simulink model "hil2DOFArmSynergyTemplate"  (R2017a)
settings: Solver=FixedStepAuto  StartTime=0.0  StopTime=5  RelTol=1e-3
undefined symbols (not defined in the file): alpha, armDynamics, get
libraries: vrlib x4, myo_lib x3, dspstat3 x2, aerolibconvert2 x1, sldrtlib x1
settings Model: Creator=ricardog  LastModifiedBy=ricardog
settings SolverCC: AutoInsertRateTranBlk=on

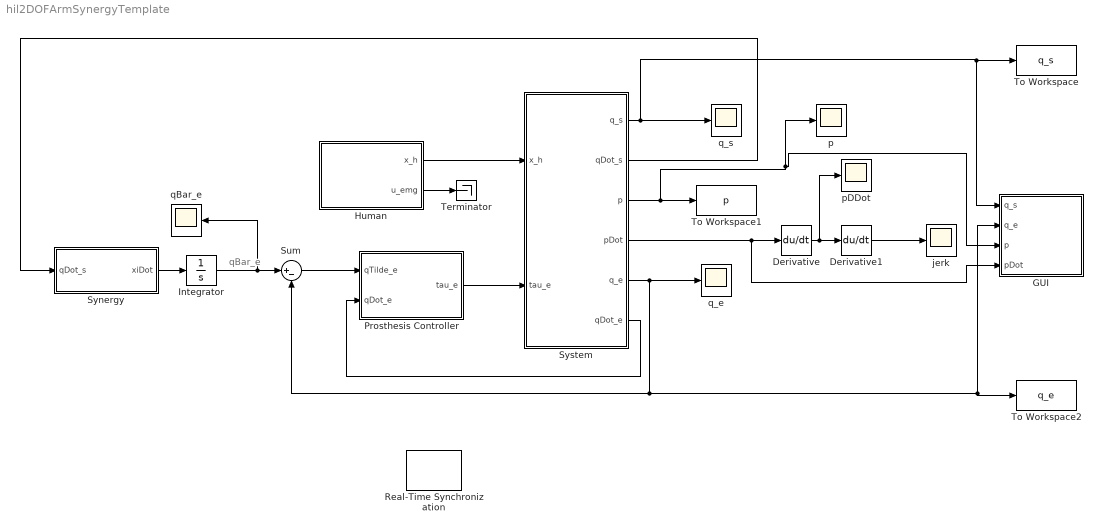
== system hil2DOFArmSynergyTemplate ==
  note: qBar_e
  Derivative : Derivative
  Derivative1 : Derivative
  GUI : Subsystem
  Human : Subsystem
  Integrator : Integrator  InitialCondition=get(armDynamics,'qInit_e')
  Prosthesis Controller : Subsystem
  Real-Time Synchronization : sldrtlib/Real-Time Synchronization  SampleTime=0.01  MaxMissedTicks=50  ShowMissedTicks=off  YieldWhenWaiting=off
  Sum : Sum  Inputs=|+-
  Synergy : Subsystem
  System : Subsystem
  Terminator : Terminator
  To Workspace : ToWorkspace  VariableName=q_s  SampleTime=-1
  To Workspace1 : ToWorkspace  VariableName=p  SampleTime=-1
  To Workspace2 : ToWorkspace  VariableName=q_e  SampleTime=-1
  jerk : Scope
  p : Scope
  pDDot : Scope
  qBar_e : Scope
  q_e : Scope
  q_s : Scope
  wires:
  Prosthesis Controller/1(tau_e) -> System/2(tau_e)
  System/6(qDot_e) -> Prosthesis Controller/2(qDot_e)
  System/5(q_e) -> q_e/1, GUI/2(q_e), To Workspace2/1, Sum/2
  Sum/1 -> Prosthesis Controller/1(qTilde_e)
  Synergy/1(xiDot) -> Integrator/1
  Integrator/1 -> qBar_e/1, Sum/1
  System/3(p) -> To Workspace1/1, GUI/3(p), p/1
  System/4(pDot) -> GUI/4(pDot), Derivative/1
  Derivative/1 -> pDDot/1, Derivative1/1
  Derivative1/1 -> jerk/1
  System/2(qDot_s) -> Synergy/1(qDot_s)
  System/1(q_s) -> GUI/1(q_s), To Workspace/1, q_s/1
  Human/1(x_h) -> System/1(x_h)
  Human/2(u_emg) -> Terminator/1

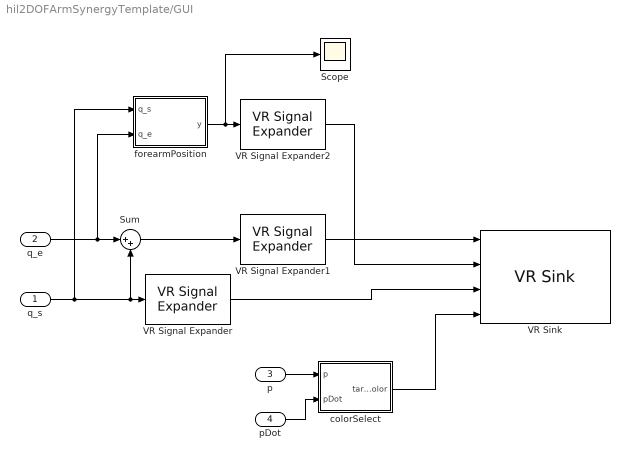
== system hil2DOFArmSynergyTemplate/GUI ==
  q_s : Inport
  q_e : Inport  Port=2
  p : Inport  Port=3
  pDot : Inport  Port=4
  Scope : Scope
  Sum : Sum  Inputs=|++
  VR Signal Expander : vrlib/VR Signal Expander  outwidth=4  outidx=[4]
      settings: SourceProductName=Simulink 3D Animation  SourceProductBaseCode=VR
  VR Signal Expander1 : vrlib/VR Signal Expander  outwidth=4  outidx=[4]
      settings: SourceProductName=Simulink 3D Animation  SourceProductBaseCode=VR
  VR Signal Expander2 : vrlib/VR Signal Expander  outwidth=3  outidx=[1 2]
      settings: SourceProductName=Simulink 3D Animation  SourceProductBaseCode=VR
  VR Sink : vrlib/VR Sink  InstantiateOnLoad=on  SampleTime=0.1  ViewEnable=on  RemoteChange=off  RemoteView=off  FieldsWritten=Forearm.rotation.4.1.1.double#Forearm.translation.3.1.1.double#UpperArm.rotation.4.1.1.double#EndTarget_material.diffuseColor.3.1.1.double  WorldFileName=C:\Users\ricardog\Documents\Workspace\HRSC_FW\GUI\armTargetsGUI.wrl  AutoView=on  VideoDimensions=[]  AllowVariableSize=off  FigureProperties="{'Position', 'Name', 'Viewpoint', 'CameraBound', 'CameraDirection', 'CameraPosition', 'CameraUpVector', 'ZoomFactor', 'Antialiasing', 'Headlight', 'Lighting', 'NavPanel', 'Sound', 'StatusBar', 'Stereo3D', 'Stereo3DCameraOffset', 'Stereo3DHIT', 'ToolBar', 'Textures', 'Transparency', 'Triad', 'Wireframe', 'NavZones', 'NavMode', 'NavSpeed', 'CaptureFileFormat', 'CaptureFileName', 'Record2DCompressMethod', 'Record2DCompressQuality', 'Record2D', 'Record2DFileName', 'Record2DFPS'; [5.8000000000000007e+00   9.1799999999999955e+01   6.8880000000000007e+02   4.7160000000000002e+02], '', 'Side view', 'on', [0.0000000000000000e+00   0.0000000000000000e+00  -1.0000000000000000e+00], [0.0000000000000000e+00   0.0000000000000000e+00   0.0000000000000000e+00], [0.0000000000000000e+00   1.0000000000000000e+00   0.0000000000000000e+00], [1.0000000000000000e+00], 'on', 'on', 'on', 'halfbar', 'on', 'on', 'off', [1.0000000149011612e-01], [0.0000000000000000e+00], 'on', 'on', 'on', 'none', 'off', 'off', 'examine', 'normal', 'tif', '%f_anim_%n.tif', 'auto', [7.5000000000000000e+01], 'off', '%f_anim_%n.avi', 'auto'}"
      settings: SourceProductBaseCode=VR
  colorSelect : MATLAB Function  TreatAsAtomicUnit=on
  forearmPosition : MATLAB Function  TreatAsAtomicUnit=on
  wires:
  q_s/1 -> Sum/2, VR Signal Expander/1, forearmPosition/1(q_s)
  forearmPosition/1(y) -> Scope/1, VR Signal Expander2/1
  Sum/1 -> VR Signal Expander1/1
  q_e/1 -> forearmPosition/2(q_e), Sum/1
  VR Signal Expander1/1 -> VR Sink/1
  VR Signal Expander2/1 -> VR Sink/2
  VR Signal Expander/1 -> VR Sink/3
  p/1 -> colorSelect/1(p)
  pDot/1 -> colorSelect/2(pDot)
  colorSelect/1(targetColor) -> VR Sink/4

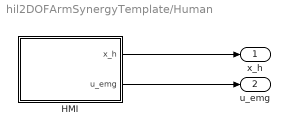
== system hil2DOFArmSynergyTemplate/Human ==
  HMI : Subsystem
  x_h : Outport
  u_emg : Outport  Port=2
  wires:
  HMI/1(x_h) -> x_h/1
  HMI/2(u_emg) -> u_emg/1

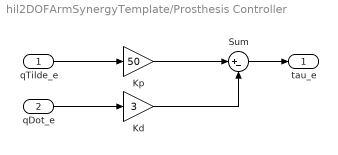
== system hil2DOFArmSynergyTemplate/Prosthesis Controller ==
  qTilde_e : Inport
  qDot_e : Inport  Port=2
  Kd : Gain  Gain=3
  Kp : Gain  Gain=50
  Sum : Sum  Inputs=|+-
  tau_e : Outport
  wires:
  qTilde_e/1 -> Kp/1
  qDot_e/1 -> Kd/1
  Kp/1 -> Sum/1
  Kd/1 -> Sum/2
  Sum/1 -> tau_e/1

== system hil2DOFArmSynergyTemplate/Synergy ==
  qDot_s : Inport
  alpha : Gain  Gain=alpha
  xiDot : Outport
  wires:
  qDot_s/1 -> alpha/1
  alpha/1 -> xiDot/1

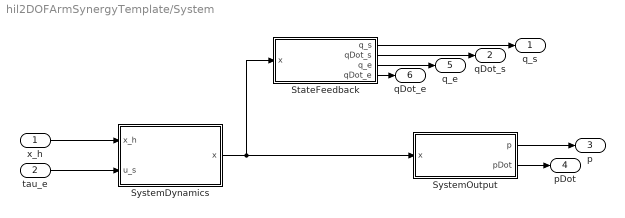
== system hil2DOFArmSynergyTemplate/System ==
  x_h : Inport
  tau_e : Inport  Port=2
  StateFeedback : Subsystem
  SystemDynamics : Subsystem
  SystemOutput : Subsystem
  q_s : Outport
  qDot_s : Outport  Port=2
  p : Outport  Port=3
  pDot : Outport  Port=4
  q_e : Outport  Port=5
  qDot_e : Outport  Port=6
  wires:
  SystemDynamics/1(x) -> StateFeedback/1(x), SystemOutput/1(x)
  SystemOutput/1(p) -> p/1
  x_h/1 -> SystemDynamics/1(x_h)
  tau_e/1 -> SystemDynamics/2(u_s)
  SystemOutput/2(pDot) -> pDot/1
  StateFeedback/1(q_s) -> q_s/1
  StateFeedback/3(q_e) -> q_e/1
  StateFeedback/2(qDot_s) -> qDot_s/1
  StateFeedback/4(qDot_e) -> qDot_e/1

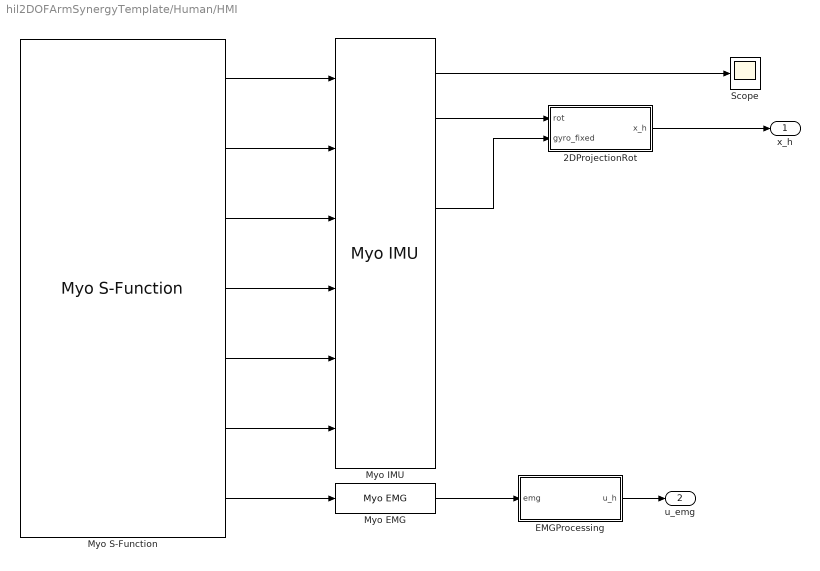
== system hil2DOFArmSynergyTemplate/Human/HMI ==
  2DProjectionRot : Subsystem
  EMGProcessing : Subsystem
  Myo EMG : myo_lib/Myo EMG
  Myo IMU : myo_lib/Myo IMU
  Myo S-Function : myo_lib/Myo S-Function  emgEnabled=1  countMyos=1
  Scope : Scope
  x_h : Outport
  u_emg : Outport  Port=2
  wires:
  Myo S-Function/3 -> Myo IMU/3
  Myo S-Function/7 -> Myo EMG/1
  Myo S-Function/4 -> Myo IMU/4
  Myo S-Function/5 -> Myo IMU/5
  Myo S-Function/2 -> Myo IMU/2
  Myo S-Function/1 -> Myo IMU/1
  Myo S-Function/6 -> Myo IMU/6
  Myo EMG/1 -> EMGProcessing/1(emg)
  EMGProcessing/1(u_h) -> u_emg/1
  Myo IMU/1 -> Scope/1
  2DProjectionRot/1(x_h) -> x_h/1
  Myo IMU/2 -> 2DProjectionRot/1(rot)
  Myo IMU/4 -> 2DProjectionRot/2(gyro_fixed)

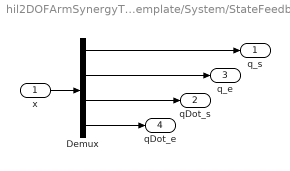
== system hil2DOFArmSynergyTemplate/System/StateFeedback ==
  x : Inport
  Demux : Demux
  q_s : Outport
  qDot_s : Outport  Port=2
  q_e : Outport  Port=3
  qDot_e : Outport  Port=4
  wires:
  x/1 -> Demux/1
  Demux/1 -> q_s/1
  Demux/3 -> qDot_s/1
  Demux/4 -> qDot_e/1
  Demux/2 -> q_e/1

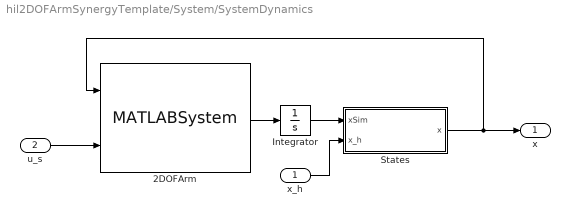
== system hil2DOFArmSynergyTemplate/System/SystemDynamics ==
  x_h : Inport
  u_s : Inport  Port=2
  2DOFArm : MATLABSystem  System=armDynamics  kS=0  kE=0  dS=-1.2  dE=-1.2  lA=0.31  lF=0.34  mA=1.93  mF=1.52  q0=[ 0; pi/2 ]  qInit_s=pi/8  qInit_e=7*pi/8  qInit=[ pi/8; 7*pi/8 ]  qDotInit=[ 0; 0 ]  SimulateUsing=Code generation
      mask Type: armDynamics
      mask Display:
      | disp('armDynamics');
      | port_label('input',1,'x');
      | port_label('input',2,'u');
      | port_label('output',1,'xDot');
  Integrator : Integrator  InitialCondition=[get(armDynamics,'qInit');get(armDynamics,'qDotInit')]  UpperSaturationLimit=100  LowerSaturationLimit=-100
  States : Subsystem
  x : Outport
  wires:
  u_s/1 -> 2DOFArm/2
  2DOFArm/1 -> Integrator/1
  Integrator/1 -> States/1(xSim)
  x_h/1 -> States/2(x_h)
  States/1(x) -> 2DOFArm/1, x/1

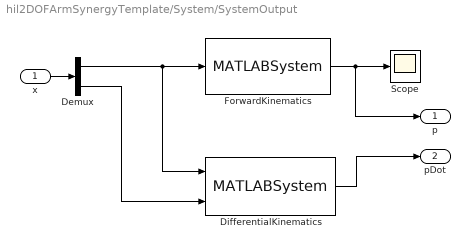
== system hil2DOFArmSynergyTemplate/System/SystemOutput ==
  x : Inport
  Demux : Demux  Outputs=2
  DifferentialKinematics : MATLABSystem  System=armDiffK  SimulateUsing=Code generation
      mask Type: armDiffK
      mask Display:
      | disp('armDiffK');
      | port_label('input',1,'q');
      | port_label('input',2,'qDot');
      | port_label('output',1,'vHand');
  ForwardKinematics : MATLABSystem  System=armFK  SimulateUsing=Code generation
      mask Type: armFK
      mask Display:
      | disp('armFK');
      | port_label('input',1,'q');
      | port_label('output',1,'xHand');
  Scope : Scope
  p : Outport
  pDot : Outport  Port=2
  wires:
  x/1 -> Demux/1
  Demux/1 -> DifferentialKinematics/1, ForwardKinematics/1
  Demux/2 -> DifferentialKinematics/2
  DifferentialKinematics/1 -> pDot/1
  ForwardKinematics/1 -> p/1, Scope/1

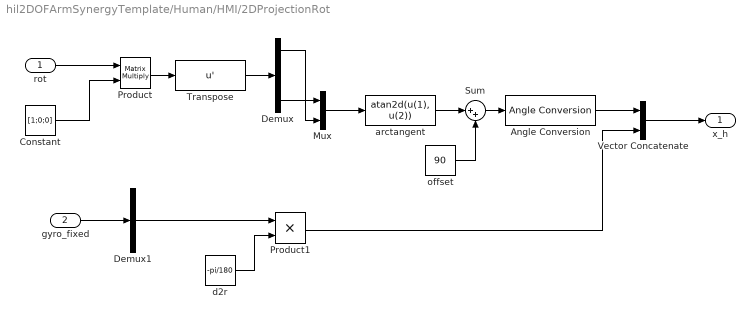
== system hil2DOFArmSynergyTemplate/Human/HMI/2DProjectionRot ==
  rot : Inport
  gyro_fixed : Inport  Port=2
  Angle Conversion : aerolibconvert2/Angle Conversion  IU=deg  OU=rad
  Constant : Constant  Value=[1;0;0]  VectorParams1D=off
  Demux : Demux  Outputs=3
  Demux1 : Demux  Outputs=3
  Mux : Mux  Inputs=2
  Product : Product  Multiplication=Matrix(*)
  Product1 : Product
  Sum : Sum  Inputs=|++
  Transpose : MATLABFcn  MATLABFcn=u'  Output1D=off
  Vector Concatenate : Concatenate
  arctangent : MATLABFcn  MATLABFcn=atan2d(u(1), u(2))
  d2r : Constant  Value=-pi/180
  offset : Constant  Value=90
  x_h : Outport
  wires:
  rot/1 -> Product/1
  Product/1 -> Transpose/1
  Constant/1 -> Product/2
  Transpose/1 -> Demux/1
  Mux/1 -> arctangent/1
  Demux/1 -> Mux/2
  Demux/3 -> Mux/1
  Vector Concatenate/1 -> x_h/1
  gyro_fixed/1 -> Demux1/1
  arctangent/1 -> Sum/1
  offset/1 -> Sum/2
  Sum/1 -> Angle Conversion/1
  Angle Conversion/1 -> Vector Concatenate/1
  Demux1/2 -> Product1/1
  d2r/1 -> Product1/2
  Product1/1 -> Vector Concatenate/2

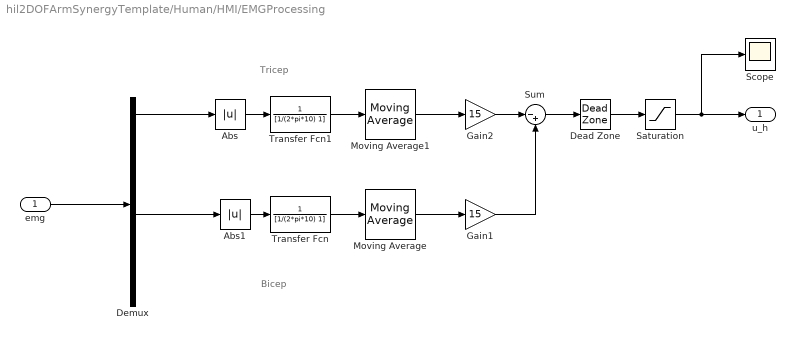
== system hil2DOFArmSynergyTemplate/Human/HMI/EMGProcessing ==
  note: Tricep
  note: Bicep
  emg : Inport
  Abs : Abs
  Abs1 : Abs
  Dead Zone : DeadZone  LowerValue=-0.7  UpperValue=0.7  SaturateOnIntegerOverflow=on
  Demux : Demux  Outputs=8
  Gain1 : Gain  Gain=15
  Gain2 : Gain  Gain=15
  Moving Average : dspstat3/Moving Average  Method=Sliding window  SpecifyWindowLength=on  WindowLength=1000  ForgettingFactor=0.9  SimulateUsing=Code generation
  Moving Average1 : dspstat3/Moving Average  Method=Sliding window  SpecifyWindowLength=on  WindowLength=1000  ForgettingFactor=0.9  SimulateUsing=Code generation
  Saturation : Saturate  UpperLimit=3  LowerLimit=-3
  Scope : Scope
  Sum : Sum  Inputs=|-+
  Transfer Fcn : TransferFcn  Denominator=[1/(2*pi*10) 1]
  Transfer Fcn1 : TransferFcn  Denominator=[1/(2*pi*10) 1]
  u_h : Outport
  wires:
  Transfer Fcn/1 -> Moving Average/1
  Moving Average/1 -> Gain1/1
  Moving Average1/1 -> Gain2/1
  Demux/5 -> Abs1/1
  Demux/1 -> Abs/1
  Abs1/1 -> Transfer Fcn/1
  Transfer Fcn1/1 -> Moving Average1/1
  Abs/1 -> Transfer Fcn1/1
  emg/1 -> Demux/1
  Gain1/1 -> Sum/2
  Gain2/1 -> Sum/1
  Saturation/1 -> Scope/1, u_h/1
  Sum/1 -> Dead Zone/1
  Dead Zone/1 -> Saturation/1

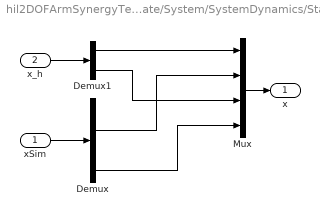
== system hil2DOFArmSynergyTemplate/System/SystemDynamics/States ==
  xSim : Inport
  x_h : Inport  Port=2
  Demux : Demux
  Demux1 : Demux  Outputs=2
  Mux : Mux
  x : Outport
  wires:
  xSim/1 -> Demux/1
  x_h/1 -> Demux1/1
  Mux/1 -> x/1
  Demux1/1 -> Mux/1
  Demux1/2 -> Mux/3
  Demux/2 -> Mux/2
  Demux/4 -> Mux/4

== matlab function hil2DOFArmSynergyTemplate/GUI/colorSelect ==
  data: p input; targetColor output; pDot input
function targetColor = fcn(p,pDot)
p_f = [0.5969;-0.0670];   % Desired end position
pNorm = norm(p-p_f);
pDotNorm = norm(pDot);
if(pNorm<0.01 && pDotNorm<0.1)
    R = 0;
    G = 1;
    B = 0;
else
    R = 0;
    G = 0;
    B = 1;
end
targetColor = [R;G;B];

== matlab function hil2DOFArmSynergyTemplate/GUI/forearmPosition ==
  data: q_s input; y output; q_e input
function y = fcn(q_s,q_e)
lA = get(armDynamics,'lA');
lF = get(armDynamics,'lF');
% xArm = (lA+(1/2)*lF)*sin(q);
% yArm = -(lA+(1/2)*lF)*cos(q);
xArm = lA*sin(q_s)+(1/2)*lF*sin(q_s+q_e);
yArm = -lA*cos(q_s)-(1/2)*lF*cos(q_s+q_e);
% xArm = lA*sin(q_s);
% yArm = -lA*cos(q_s);
% xArm = 0;
% yArm = 0;
y = [xArm;yArm];
